simulink model "switch_control"  (Simulink 6.3)
settings: Solver=FixedStepDiscrete  StartTime=0.0  StopTime=10.0  RelTol=1e-3
InitFcn:
  | %% DSPBuilder Start
  | alt_dspbuilder_update_model(bdroot)
  | %% DSPBuilder End
libraries: allblocks_alteradspbuilder2 x11
settings Model: LastModifiedBy=gnixon  StrictBusMsg=None
settings DataIOCC: SignalLoggingName=sigsOut
settings OptimizationCC: BlockReduction=off  BooleanDataType=off  InlineInvariantSignals=on
settings DebuggingCC: SolverPrmCheckMsg=none
settings HardwareCC: TargetUnknown=on

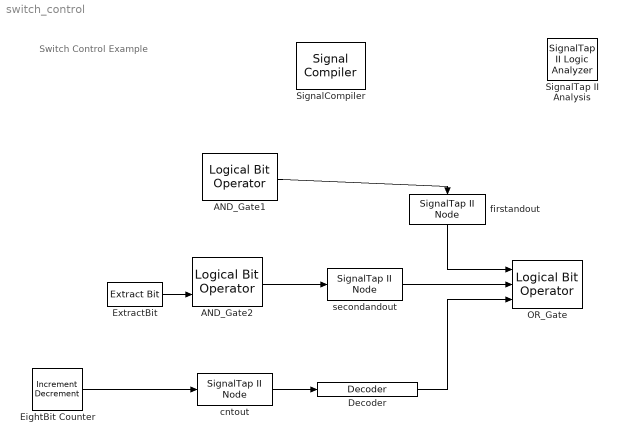
== system switch_control ==
  note: Switch Control Example
  AND_Gate1 : allblocks_alteradspbuilder2/Logical Bit Operator  LogicalOperator=AND  user_inputs=2
  AND_Gate2 : allblocks_alteradspbuilder2/Logical Bit Operator  LogicalOperator=AND  user_inputs=2
  Decoder : allblocks_alteradspbuilder2/Decoder  BusType=Unsigned Integer  bwl=8  bwr=0  registered=off  value=0
  EightBit Counter : allblocks_alteradspbuilder2/Increment Decrement  BusType=Unsigned Integer  bwl=8  bwr=0  SpecifyClock=off  clr_value=0  direction=Increment  phase_selection=1  use_ena=off  use_sclr=off
  ExtractBit : allblocks_alteradspbuilder2/Extract Bit  BusType=Signed Fractional  bwl=8  bwr=0  bitToSelect=1
  OR_Gate : allblocks_alteradspbuilder2/Logical Bit Operator  LogicalOperator=OR  user_inputs=3
  SignalCompiler : allblocks_alteradspbuilder2/Signal Compiler  DeviceFamily=DSP Board  DeviceName=AUTO  EnableSignalTap=on  SignalTapDepth=128  UseBoardBlock=off  StpUseDefaultClock=on  StpClock=clock
  SignalTap II Analysis : allblocks_alteradspbuilder2/SignalTap II Logic Analyzer
  cntout : allblocks_alteradspbuilder2/SignalTap II Node  id=0
  firstandout : allblocks_alteradspbuilder2/SignalTap II Node  Orientation=down  id=1
  secondandout : allblocks_alteradspbuilder2/SignalTap II Node  id=2
  wires:
  EightBit Counter/1 -> cntout/1
  AND_Gate2/1 -> secondandout/1
  Decoder/1 -> OR_Gate/3
  cntout/1 -> Decoder/1
  AND_Gate1/1 -> firstandout/1
  firstandout/1 -> OR_Gate/1
  secondandout/1 -> OR_Gate/2
  ExtractBit/1 -> AND_Gate2/2
